simulink model "h16k_ver112c_1500"  (R2012b)
settings: Solver=VariableStepDiscrete  SolverMode=SingleTasking  StartTime=0.0  StopTime=128000  RelTol=1e-3
undefined symbols (not defined in the file or in its folder): sfp
libraries: xbsIndex_r4 x3386, dspsigops x32, casper_library_misc x23, monroe_library x8, simulink x7, xps_library x6
(part 2 of 28)

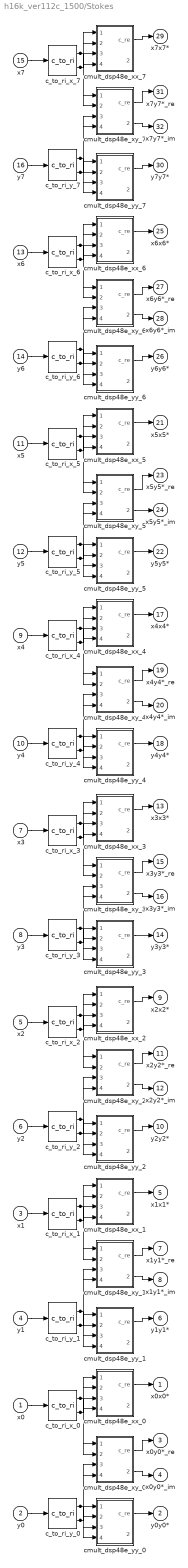
== system h16k_ver112c_1500/Stokes ==
  x0 : Inport
  y0 : Inport  Port=2
  x1 : Inport  Port=3
  y1 : Inport  Port=4
  x2 : Inport  Port=5
  y2 : Inport  Port=6
  x3 : Inport  Port=7
  y3 : Inport  Port=8
  x4 : Inport  Port=9
  y4 : Inport  Port=10
  x5 : Inport  Port=11
  y5 : Inport  Port=12
  x6 : Inport  Port=13
  y6 : Inport  Port=14
  x7 : Inport  Port=15
  y7 : Inport  Port=16
  c_to_ri_x_{0..7} (8 alike) : casper_library_misc/c_to_ri  n_bits=18  bin_pt=0
      settings: AttributesFormatString=18_0 r/i
  c_to_ri_y_{0..7} (8 alike) : casper_library_misc/c_to_ri  n_bits=18  bin_pt=0
      settings: AttributesFormatString=18_0 r/i
  cmult_dsp48e_xx_0 : Subsystem  AncestorBlock=casper_library_multipliers/cmult_dsp48e  mask(cmult_dsp48e){n_bits_a=18, bin_pt_a=0, n_bits_b=18, bin_pt_b=0, conjugated=on, full_precision=on, n_bits_c=37, bin_pt_c=34, quantization=Truncate, overflow=Wrap, cast_latency=0}
      mask prompts: n_bits_a "Bit width 'a'"; bin_pt_a "Binary point 'a'"; n_bits_b "Bit width 'b'"; bin_pt_b "Binary point 'b'"; conjugated "Conjugate"; full_precision "Full precision"; n_bits_c "Bit width out"; bin_pt_c "Binary point out"; cast_latency "Cast Latency"
      mask help:
      | Multiplies two complex numbers using 4 DSP48Es.
      | Conjugation is optional.
      |
      | Re{a} and Im{a} can be up to 25 bits.
      | Re{b} and Im{b} can be up to 18 bits.
      mask init:
      | cmult_dsp48e_init(gcb, ...
      |     'n_bits_a', n_bits_a, ...
      |     'bin_pt_a', bin_pt_a, ...
      |     'n_bits_b', n_bits_b, ...
      |     'bin_pt_b', bin_pt_b, ...
      |     'conjugated', conjugated, ...
      |     'full_precision', full_precision, ...
      |     'n_bits_c', n_bits_c, ...
      |     'bin_pt_c', bin_pt_c, ...
      |     'quantization', quantization, ...
      |     'overflow', overflow, ...
      |     'cast_latency', cast_latency);
      settings: AttributesFormatString=|
      | 18_0 * 18_0 ==> 37_0
      | Latency=4
      mask Callback full_precision:
      | full_precision = get_param(gcb, 'full_precision');
      | 
      | if strcmp(full_precision, 'on'),
      |     not_full_precision = 'off';
      | else
      |     not_full_precision = 'on';
      | end
      | 
      | set_param_state(gcb, 'n_bits_c', not_full_precision);
      | set_param_state(gcb, 'bin_pt_c', not_full_precision);
      | set_param_state(gcb, 'quantization', not_full_precision);
      | set_param_state(gcb, 'overflow', not_full_precision);
      | set_param_state(gcb, 'cast_latency', not_full_precision);
      mask TypeOptions quantization: Truncate | Round  (unbiased: +/- Inf) | Round  (unbiased: Even Values)
      mask TypeOptions overflow: Wrap | Saturate | Flag as error
  cmult_dsp48e_xx_1 : Subsystem  AncestorBlock=casper_library_multipliers/cmult_dsp48e  mask(cmult_dsp48e){n_bits_a=18, bin_pt_a=0, n_bits_b=18, bin_pt_b=0, conjugated=on, full_precision=on, n_bits_c=37, bin_pt_c=34, quantization=Truncate, overflow=Wrap, cast_latency=0}
      mask prompts: n_bits_a "Bit width 'a'"; bin_pt_a "Binary point 'a'"; n_bits_b "Bit width 'b'"; bin_pt_b "Binary point 'b'"; conjugated "Conjugate"; full_precision "Full precision"; n_bits_c "Bit width out"; bin_pt_c "Binary point out"; cast_latency "Cast Latency"
      mask help:
      | Multiplies two complex numbers using 4 DSP48Es.
      | Conjugation is optional.
      |
      | Re{a} and Im{a} can be up to 25 bits.
      | Re{b} and Im{b} can be up to 18 bits.
      mask init: same as h16k_ver112c_1500/Stokes/cmult_dsp48e_xx_0
      settings: AttributesFormatString=|
      | 18_0 * 18_0 ==> 37_0
      | Latency=4
      mask Callback full_precision:
      | full_precision = get_param(gcb, 'full_precision');
      | 
      | if strcmp(full_precision, 'on'),
      |     not_full_precision = 'off';
      | else
      |     not_full_precision = 'on';
      | end
      | 
      | set_param_state(gcb, 'n_bits_c', not_full_precision);
      | set_param_state(gcb, 'bin_pt_c', not_full_precision);
      | set_param_state(gcb, 'quantization', not_full_precision);
      | set_param_state(gcb, 'overflow', not_full_precision);
      | set_param_state(gcb, 'cast_latency', not_full_precision);
      mask TypeOptions quantization: Truncate | Round  (unbiased: +/- Inf) | Round  (unbiased: Even Values)
      mask TypeOptions overflow: Wrap | Saturate | Flag as error
  cmult_dsp48e_xx_2 : Subsystem  AncestorBlock=casper_library_multipliers/cmult_dsp48e  mask(cmult_dsp48e){n_bits_a=18, bin_pt_a=0, n_bits_b=18, bin_pt_b=0, conjugated=on, full_precision=on, n_bits_c=37, bin_pt_c=34, quantization=Truncate, overflow=Wrap, cast_latency=0}
      mask prompts: n_bits_a "Bit width 'a'"; bin_pt_a "Binary point 'a'"; n_bits_b "Bit width 'b'"; bin_pt_b "Binary point 'b'"; conjugated "Conjugate"; full_precision "Full precision"; n_bits_c "Bit width out"; bin_pt_c "Binary point out"; cast_latency "Cast Latency"
      mask help:
      | Multiplies two complex numbers using 4 DSP48Es.
      | Conjugation is optional.
      |
      | Re{a} and Im{a} can be up to 25 bits.
      | Re{b} and Im{b} can be up to 18 bits.
      mask init: same as h16k_ver112c_1500/Stokes/cmult_dsp48e_xx_0
      settings: AttributesFormatString=|
      | 18_0 * 18_0 ==> 37_0
      | Latency=4
      mask Callback full_precision:
      | full_precision = get_param(gcb, 'full_precision');
      | 
      | if strcmp(full_precision, 'on'),
      |     not_full_precision = 'off';
      | else
      |     not_full_precision = 'on';
      | end
      | 
      | set_param_state(gcb, 'n_bits_c', not_full_precision);
      | set_param_state(gcb, 'bin_pt_c', not_full_precision);
      | set_param_state(gcb, 'quantization', not_full_precision);
      | set_param_state(gcb, 'overflow', not_full_precision);
      | set_param_state(gcb, 'cast_latency', not_full_precision);
      mask TypeOptions quantization: Truncate | Round  (unbiased: +/- Inf) | Round  (unbiased: Even Values)
      mask TypeOptions overflow: Wrap | Saturate | Flag as error
  cmult_dsp48e_xx_3 : Subsystem  AncestorBlock=casper_library_multipliers/cmult_dsp48e  mask(cmult_dsp48e){n_bits_a=18, bin_pt_a=0, n_bits_b=18, bin_pt_b=0, conjugated=on, full_precision=on, n_bits_c=37, bin_pt_c=34, quantization=Truncate, overflow=Wrap, cast_latency=0}
      mask prompts: n_bits_a "Bit width 'a'"; bin_pt_a "Binary point 'a'"; n_bits_b "Bit width 'b'"; bin_pt_b "Binary point 'b'"; conjugated "Conjugate"; full_precision "Full precision"; n_bits_c "Bit width out"; bin_pt_c "Binary point out"; cast_latency "Cast Latency"
      mask help:
      | Multiplies two complex numbers using 4 DSP48Es.
      | Conjugation is optional.
      |
      | Re{a} and Im{a} can be up to 25 bits.
      | Re{b} and Im{b} can be up to 18 bits.
      mask init: same as h16k_ver112c_1500/Stokes/cmult_dsp48e_xx_0
      settings: AttributesFormatString=|
      | 18_0 * 18_0 ==> 37_0
      | Latency=4
      mask Callback full_precision:
      | full_precision = get_param(gcb, 'full_precision');
      | 
      | if strcmp(full_precision, 'on'),
      |     not_full_precision = 'off';
      | else
      |     not_full_precision = 'on';
      | end
      | 
      | set_param_state(gcb, 'n_bits_c', not_full_precision);
      | set_param_state(gcb, 'bin_pt_c', not_full_precision);
      | set_param_state(gcb, 'quantization', not_full_precision);
      | set_param_state(gcb, 'overflow', not_full_precision);
      | set_param_state(gcb, 'cast_latency', not_full_precision);
      mask TypeOptions quantization: Truncate | Round  (unbiased: +/- Inf) | Round  (unbiased: Even Values)
      mask TypeOptions overflow: Wrap | Saturate | Flag as error
  cmult_dsp48e_xx_4 : Subsystem  AncestorBlock=casper_library_multipliers/cmult_dsp48e  mask(cmult_dsp48e){n_bits_a=18, bin_pt_a=0, n_bits_b=18, bin_pt_b=0, conjugated=on, full_precision=on, n_bits_c=37, bin_pt_c=34, quantization=Truncate, overflow=Wrap, cast_latency=0}
      mask prompts: n_bits_a "Bit width 'a'"; bin_pt_a "Binary point 'a'"; n_bits_b "Bit width 'b'"; bin_pt_b "Binary point 'b'"; conjugated "Conjugate"; full_precision "Full precision"; n_bits_c "Bit width out"; bin_pt_c "Binary point out"; cast_latency "Cast Latency"
      mask help:
      | Multiplies two complex numbers using 4 DSP48Es.
      | Conjugation is optional.
      |
      | Re{a} and Im{a} can be up to 25 bits.
      | Re{b} and Im{b} can be up to 18 bits.
      mask init: same as h16k_ver112c_1500/Stokes/cmult_dsp48e_xx_0
      settings: AttributesFormatString=|
      | 18_0 * 18_0 ==> 37_0
      | Latency=4
      mask Callback full_precision:
      | full_precision = get_param(gcb, 'full_precision');
      | 
      | if strcmp(full_precision, 'on'),
      |     not_full_precision = 'off';
      | else
      |     not_full_precision = 'on';
      | end
      | 
      | set_param_state(gcb, 'n_bits_c', not_full_precision);
      | set_param_state(gcb, 'bin_pt_c', not_full_precision);
      | set_param_state(gcb, 'quantization', not_full_precision);
      | set_param_state(gcb, 'overflow', not_full_precision);
      | set_param_state(gcb, 'cast_latency', not_full_precision);
      mask TypeOptions quantization: Truncate | Round  (unbiased: +/- Inf) | Round  (unbiased: Even Values)
      mask TypeOptions overflow: Wrap | Saturate | Flag as error
  cmult_dsp48e_xx_5 : Subsystem  AncestorBlock=casper_library_multipliers/cmult_dsp48e  mask(cmult_dsp48e){n_bits_a=18, bin_pt_a=0, n_bits_b=18, bin_pt_b=0, conjugated=on, full_precision=on, n_bits_c=37, bin_pt_c=34, quantization=Truncate, overflow=Wrap, cast_latency=0}
      mask prompts: n_bits_a "Bit width 'a'"; bin_pt_a "Binary point 'a'"; n_bits_b "Bit width 'b'"; bin_pt_b "Binary point 'b'"; conjugated "Conjugate"; full_precision "Full precision"; n_bits_c "Bit width out"; bin_pt_c "Binary point out"; cast_latency "Cast Latency"
      mask help:
      | Multiplies two complex numbers using 4 DSP48Es.
      | Conjugation is optional.
      |
      | Re{a} and Im{a} can be up to 25 bits.
      | Re{b} and Im{b} can be up to 18 bits.
      mask init: same as h16k_ver112c_1500/Stokes/cmult_dsp48e_xx_0
      settings: AttributesFormatString=|
      | 18_0 * 18_0 ==> 37_0
      | Latency=4
      mask Callback full_precision:
      | full_precision = get_param(gcb, 'full_precision');
      | 
      | if strcmp(full_precision, 'on'),
      |     not_full_precision = 'off';
      | else
      |     not_full_precision = 'on';
      | end
      | 
      | set_param_state(gcb, 'n_bits_c', not_full_precision);
      | set_param_state(gcb, 'bin_pt_c', not_full_precision);
      | set_param_state(gcb, 'quantization', not_full_precision);
      | set_param_state(gcb, 'overflow', not_full_precision);
      | set_param_state(gcb, 'cast_latency', not_full_precision);
      mask TypeOptions quantization: Truncate | Round  (unbiased: +/- Inf) | Round  (unbiased: Even Values)
      mask TypeOptions overflow: Wrap | Saturate | Flag as error
  cmult_dsp48e_xx_6 : Subsystem  AncestorBlock=casper_library_multipliers/cmult_dsp48e  mask(cmult_dsp48e){n_bits_a=18, bin_pt_a=0, n_bits_b=18, bin_pt_b=0, conjugated=on, full_precision=on, n_bits_c=37, bin_pt_c=34, quantization=Truncate, overflow=Wrap, cast_latency=0}
      mask prompts: n_bits_a "Bit width 'a'"; bin_pt_a "Binary point 'a'"; n_bits_b "Bit width 'b'"; bin_pt_b "Binary point 'b'"; conjugated "Conjugate"; full_precision "Full precision"; n_bits_c "Bit width out"; bin_pt_c "Binary point out"; cast_latency "Cast Latency"
      mask help:
      | Multiplies two complex numbers using 4 DSP48Es.
      | Conjugation is optional.
      |
      | Re{a} and Im{a} can be up to 25 bits.
      | Re{b} and Im{b} can be up to 18 bits.
      mask init: same as h16k_ver112c_1500/Stokes/cmult_dsp48e_xx_0
      settings: AttributesFormatString=|
      | 18_0 * 18_0 ==> 37_0
      | Latency=4
      mask Callback full_precision:
      | full_precision = get_param(gcb, 'full_precision');
      | 
      | if strcmp(full_precision, 'on'),
      |     not_full_precision = 'off';
      | else
      |     not_full_precision = 'on';
      | end
      | 
      | set_param_state(gcb, 'n_bits_c', not_full_precision);
      | set_param_state(gcb, 'bin_pt_c', not_full_precision);
      | set_param_state(gcb, 'quantization', not_full_precision);
      | set_param_state(gcb, 'overflow', not_full_precision);
      | set_param_state(gcb, 'cast_latency', not_full_precision);
      mask TypeOptions quantization: Truncate | Round  (unbiased: +/- Inf) | Round  (unbiased: Even Values)
      mask TypeOptions overflow: Wrap | Saturate | Flag as error
  cmult_dsp48e_xx_7 : Subsystem  AncestorBlock=casper_library_multipliers/cmult_dsp48e  mask(cmult_dsp48e){n_bits_a=18, bin_pt_a=0, n_bits_b=18, bin_pt_b=0, conjugated=on, full_precision=on, n_bits_c=37, bin_pt_c=34, quantization=Truncate, overflow=Wrap, cast_latency=0}
      mask prompts: n_bits_a "Bit width 'a'"; bin_pt_a "Binary point 'a'"; n_bits_b "Bit width 'b'"; bin_pt_b "Binary point 'b'"; conjugated "Conjugate"; full_precision "Full precision"; n_bits_c "Bit width out"; bin_pt_c "Binary point out"; cast_latency "Cast Latency"
      mask help:
      | Multiplies two complex numbers using 4 DSP48Es.
      | Conjugation is optional.
      |
      | Re{a} and Im{a} can be up to 25 bits.
      | Re{b} and Im{b} can be up to 18 bits.
      mask init: same as h16k_ver112c_1500/Stokes/cmult_dsp48e_xx_0
      settings: AttributesFormatString=|
      | 18_0 * 18_0 ==> 37_0
      | Latency=4
      mask Callback full_precision:
      | full_precision = get_param(gcb, 'full_precision');
      | 
      | if strcmp(full_precision, 'on'),
      |     not_full_precision = 'off';
      | else
      |     not_full_precision = 'on';
      | end
      | 
      | set_param_state(gcb, 'n_bits_c', not_full_precision);
      | set_param_state(gcb, 'bin_pt_c', not_full_precision);
      | set_param_state(gcb, 'quantization', not_full_precision);
      | set_param_state(gcb, 'overflow', not_full_precision);
      | set_param_state(gcb, 'cast_latency', not_full_precision);
      mask TypeOptions quantization: Truncate | Round  (unbiased: +/- Inf) | Round  (unbiased: Even Values)
      mask TypeOptions overflow: Wrap | Saturate | Flag as error
  cmult_dsp48e_xy_0 : Subsystem  AncestorBlock=casper_library_multipliers/cmult_dsp48e  mask(cmult_dsp48e){n_bits_a=18, bin_pt_a=0, n_bits_b=18, bin_pt_b=0, conjugated=on, full_precision=on, n_bits_c=37, bin_pt_c=34, quantization=Truncate, overflow=Wrap, cast_latency=0}
      mask prompts: n_bits_a "Bit width 'a'"; bin_pt_a "Binary point 'a'"; n_bits_b "Bit width 'b'"; bin_pt_b "Binary point 'b'"; conjugated "Conjugate"; full_precision "Full precision"; n_bits_c "Bit width out"; bin_pt_c "Binary point out"; cast_latency "Cast Latency"
      mask help:
      | Multiplies two complex numbers using 4 DSP48Es.
      | Conjugation is optional.
      |
      | Re{a} and Im{a} can be up to 25 bits.
      | Re{b} and Im{b} can be up to 18 bits.
      mask init: same as h16k_ver112c_1500/Stokes/cmult_dsp48e_xx_0
      settings: AttributesFormatString=|
      | 18_0 * 18_0 ==> 37_0
      | Latency=4
      mask Callback full_precision:
      | full_precision = get_param(gcb, 'full_precision');
      | 
      | if strcmp(full_precision, 'on'),
      |     not_full_precision = 'off';
      | else
      |     not_full_precision = 'on';
      | end
      | 
      | set_param_state(gcb, 'n_bits_c', not_full_precision);
      | set_param_state(gcb, 'bin_pt_c', not_full_precision);
      | set_param_state(gcb, 'quantization', not_full_precision);
      | set_param_state(gcb, 'overflow', not_full_precision);
      | set_param_state(gcb, 'cast_latency', not_full_precision);
      mask TypeOptions quantization: Truncate | Round  (unbiased: +/- Inf) | Round  (unbiased: Even Values)
      mask TypeOptions overflow: Wrap | Saturate | Flag as error
  cmult_dsp48e_xy_1 : Subsystem  AncestorBlock=casper_library_multipliers/cmult_dsp48e  mask(cmult_dsp48e){n_bits_a=18, bin_pt_a=0, n_bits_b=18, bin_pt_b=0, conjugated=on, full_precision=on, n_bits_c=37, bin_pt_c=34, quantization=Truncate, overflow=Wrap, cast_latency=0}
      mask prompts: n_bits_a "Bit width 'a'"; bin_pt_a "Binary point 'a'"; n_bits_b "Bit width 'b'"; bin_pt_b "Binary point 'b'"; conjugated "Conjugate"; full_precision "Full precision"; n_bits_c "Bit width out"; bin_pt_c "Binary point out"; cast_latency "Cast Latency"
      mask help:
      | Multiplies two complex numbers using 4 DSP48Es.
      | Conjugation is optional.
      |
      | Re{a} and Im{a} can be up to 25 bits.
      | Re{b} and Im{b} can be up to 18 bits.
      mask init: same as h16k_ver112c_1500/Stokes/cmult_dsp48e_xx_0
      settings: AttributesFormatString=|
      | 18_0 * 18_0 ==> 37_0
      | Latency=4
      mask Callback full_precision:
      | full_precision = get_param(gcb, 'full_precision');
      | 
      | if strcmp(full_precision, 'on'),
      |     not_full_precision = 'off';
      | else
      |     not_full_precision = 'on';
      | end
      | 
      | set_param_state(gcb, 'n_bits_c', not_full_precision);
      | set_param_state(gcb, 'bin_pt_c', not_full_precision);
      | set_param_state(gcb, 'quantization', not_full_precision);
      | set_param_state(gcb, 'overflow', not_full_precision);
      | set_param_state(gcb, 'cast_latency', not_full_precision);
      mask TypeOptions quantization: Truncate | Round  (unbiased: +/- Inf) | Round  (unbiased: Even Values)
      mask TypeOptions overflow: Wrap | Saturate | Flag as error
  cmult_dsp48e_xy_2 : Subsystem  AncestorBlock=casper_library_multipliers/cmult_dsp48e  mask(cmult_dsp48e){n_bits_a=18, bin_pt_a=0, n_bits_b=18, bin_pt_b=0, conjugated=on, full_precision=on, n_bits_c=37, bin_pt_c=34, quantization=Truncate, overflow=Wrap, cast_latency=0}
      mask prompts: n_bits_a "Bit width 'a'"; bin_pt_a "Binary point 'a'"; n_bits_b "Bit width 'b'"; bin_pt_b "Binary point 'b'"; conjugated "Conjugate"; full_precision "Full precision"; n_bits_c "Bit width out"; bin_pt_c "Binary point out"; cast_latency "Cast Latency"
      mask help:
      | Multiplies two complex numbers using 4 DSP48Es.
      | Conjugation is optional.
      |
      | Re{a} and Im{a} can be up to 25 bits.
      | Re{b} and Im{b} can be up to 18 bits.
      mask init: same as h16k_ver112c_1500/Stokes/cmult_dsp48e_xx_0
      settings: AttributesFormatString=|
      | 18_0 * 18_0 ==> 37_0
      | Latency=4
      mask Callback full_precision:
      | full_precision = get_param(gcb, 'full_precision');
      | 
      | if strcmp(full_precision, 'on'),
      |     not_full_precision = 'off';
      | else
      |     not_full_precision = 'on';
      | end
      | 
      | set_param_state(gcb, 'n_bits_c', not_full_precision);
      | set_param_state(gcb, 'bin_pt_c', not_full_precision);
      | set_param_state(gcb, 'quantization', not_full_precision);
      | set_param_state(gcb, 'overflow', not_full_precision);
      | set_param_state(gcb, 'cast_latency', not_full_precision);
      mask TypeOptions quantization: Truncate | Round  (unbiased: +/- Inf) | Round  (unbiased: Even Values)
      mask TypeOptions overflow: Wrap | Saturate | Flag as error
  cmult_dsp48e_xy_3 : Subsystem  AncestorBlock=casper_library_multipliers/cmult_dsp48e  mask(cmult_dsp48e){n_bits_a=18, bin_pt_a=0, n_bits_b=18, bin_pt_b=0, conjugated=on, full_precision=on, n_bits_c=37, bin_pt_c=34, quantization=Truncate, overflow=Wrap, cast_latency=0}
      mask prompts: n_bits_a "Bit width 'a'"; bin_pt_a "Binary point 'a'"; n_bits_b "Bit width 'b'"; bin_pt_b "Binary point 'b'"; conjugated "Conjugate"; full_precision "Full precision"; n_bits_c "Bit width out"; bin_pt_c "Binary point out"; cast_latency "Cast Latency"
      mask help:
      | Multiplies two complex numbers using 4 DSP48Es.
      | Conjugation is optional.
      |
      | Re{a} and Im{a} can be up to 25 bits.
      | Re{b} and Im{b} can be up to 18 bits.
      mask init: same as h16k_ver112c_1500/Stokes/cmult_dsp48e_xx_0
      settings: AttributesFormatString=|
      | 18_0 * 18_0 ==> 37_0
      | Latency=4
      mask Callback full_precision:
      | full_precision = get_param(gcb, 'full_precision');
      | 
      | if strcmp(full_precision, 'on'),
      |     not_full_precision = 'off';
      | else
      |     not_full_precision = 'on';
      | end
      | 
      | set_param_state(gcb, 'n_bits_c', not_full_precision);
      | set_param_state(gcb, 'bin_pt_c', not_full_precision);
      | set_param_state(gcb, 'quantization', not_full_precision);
      | set_param_state(gcb, 'overflow', not_full_precision);
      | set_param_state(gcb, 'cast_latency', not_full_precision);
      mask TypeOptions quantization: Truncate | Round  (unbiased: +/- Inf) | Round  (unbiased: Even Values)
      mask TypeOptions overflow: Wrap | Saturate | Flag as error
  cmult_dsp48e_xy_4 : Subsystem  AncestorBlock=casper_library_multipliers/cmult_dsp48e  mask(cmult_dsp48e){n_bits_a=18, bin_pt_a=0, n_bits_b=18, bin_pt_b=0, conjugated=on, full_precision=on, n_bits_c=37, bin_pt_c=34, quantization=Truncate, overflow=Wrap, cast_latency=0}
      mask prompts: n_bits_a "Bit width 'a'"; bin_pt_a "Binary point 'a'"; n_bits_b "Bit width 'b'"; bin_pt_b "Binary point 'b'"; conjugated "Conjugate"; full_precision "Full precision"; n_bits_c "Bit width out"; bin_pt_c "Binary point out"; cast_latency "Cast Latency"
      mask help:
      | Multiplies two complex numbers using 4 DSP48Es.
      | Conjugation is optional.
      |
      | Re{a} and Im{a} can be up to 25 bits.
      | Re{b} and Im{b} can be up to 18 bits.
      mask init: same as h16k_ver112c_1500/Stokes/cmult_dsp48e_xx_0
      settings: AttributesFormatString=|
      | 18_0 * 18_0 ==> 37_0
      | Latency=4
      mask Callback full_precision:
      | full_precision = get_param(gcb, 'full_precision');
      | 
      | if strcmp(full_precision, 'on'),
      |     not_full_precision = 'off';
      | else
      |     not_full_precision = 'on';
      | end
      | 
      | set_param_state(gcb, 'n_bits_c', not_full_precision);
      | set_param_state(gcb, 'bin_pt_c', not_full_precision);
      | set_param_state(gcb, 'quantization', not_full_precision);
      | set_param_state(gcb, 'overflow', not_full_precision);
      | set_param_state(gcb, 'cast_latency', not_full_precision);
      mask TypeOptions quantization: Truncate | Round  (unbiased: +/- Inf) | Round  (unbiased: Even Values)
      mask TypeOptions overflow: Wrap | Saturate | Flag as error
  cmult_dsp48e_xy_5 : Subsystem  AncestorBlock=casper_library_multipliers/cmult_dsp48e  mask(cmult_dsp48e){n_bits_a=18, bin_pt_a=0, n_bits_b=18, bin_pt_b=0, conjugated=on, full_precision=on, n_bits_c=37, bin_pt_c=34, quantization=Truncate, overflow=Wrap, cast_latency=0}
      mask prompts: n_bits_a "Bit width 'a'"; bin_pt_a "Binary point 'a'"; n_bits_b "Bit width 'b'"; bin_pt_b "Binary point 'b'"; conjugated "Conjugate"; full_precision "Full precision"; n_bits_c "Bit width out"; bin_pt_c "Binary point out"; cast_latency "Cast Latency"
      mask help:
      | Multiplies two complex numbers using 4 DSP48Es.
      | Conjugation is optional.
      |
      | Re{a} and Im{a} can be up to 25 bits.
      | Re{b} and Im{b} can be up to 18 bits.
      mask init: same as h16k_ver112c_1500/Stokes/cmult_dsp48e_xx_0
      settings: AttributesFormatString=|
      | 18_0 * 18_0 ==> 37_0
      | Latency=4
      mask Callback full_precision:
      | full_precision = get_param(gcb, 'full_precision');
      | 
      | if strcmp(full_precision, 'on'),
      |     not_full_precision = 'off';
      | else
      |     not_full_precision = 'on';
      | end
      | 
      | set_param_state(gcb, 'n_bits_c', not_full_precision);
      | set_param_state(gcb, 'bin_pt_c', not_full_precision);
      | set_param_state(gcb, 'quantization', not_full_precision);
      | set_param_state(gcb, 'overflow', not_full_precision);
      | set_param_state(gcb, 'cast_latency', not_full_precision);
      mask TypeOptions quantization: Truncate | Round  (unbiased: +/- Inf) | Round  (unbiased: Even Values)
      mask TypeOptions overflow: Wrap | Saturate | Flag as error
  cmult_dsp48e_xy_6 : Subsystem  AncestorBlock=casper_library_multipliers/cmult_dsp48e  mask(cmult_dsp48e){n_bits_a=18, bin_pt_a=0, n_bits_b=18, bin_pt_b=0, conjugated=on, full_precision=on, n_bits_c=37, bin_pt_c=34, quantization=Truncate, overflow=Wrap, cast_latency=0}
      mask prompts: n_bits_a "Bit width 'a'"; bin_pt_a "Binary point 'a'"; n_bits_b "Bit width 'b'"; bin_pt_b "Binary point 'b'"; conjugated "Conjugate"; full_precision "Full precision"; n_bits_c "Bit width out"; bin_pt_c "Binary point out"; cast_latency "Cast Latency"
      mask help:
      | Multiplies two complex numbers using 4 DSP48Es.
      | Conjugation is optional.
      |
      | Re{a} and Im{a} can be up to 25 bits.
      | Re{b} and Im{b} can be up to 18 bits.
      mask init: same as h16k_ver112c_1500/Stokes/cmult_dsp48e_xx_0
      settings: AttributesFormatString=|
      | 18_0 * 18_0 ==> 37_0
      | Latency=4
      mask Callback full_precision:
      | full_precision = get_param(gcb, 'full_precision');
      | 
      | if strcmp(full_precision, 'on'),
      |     not_full_precision = 'off';
      | else
      |     not_full_precision = 'on';
      | end
      | 
      | set_param_state(gcb, 'n_bits_c', not_full_precision);
      | set_param_state(gcb, 'bin_pt_c', not_full_precision);
      | set_param_state(gcb, 'quantization', not_full_precision);
      | set_param_state(gcb, 'overflow', not_full_precision);
      | set_param_state(gcb, 'cast_latency', not_full_precision);
      mask TypeOptions quantization: Truncate | Round  (unbiased: +/- Inf) | Round  (unbiased: Even Values)
      mask TypeOptions overflow: Wrap | Saturate | Flag as error
  cmult_dsp48e_xy_7 : Subsystem  AncestorBlock=casper_library_multipliers/cmult_dsp48e  mask(cmult_dsp48e){n_bits_a=18, bin_pt_a=0, n_bits_b=18, bin_pt_b=0, conjugated=on, full_precision=on, n_bits_c=37, bin_pt_c=34, quantization=Truncate, overflow=Wrap, cast_latency=0}
      mask prompts: n_bits_a "Bit width 'a'"; bin_pt_a "Binary point 'a'"; n_bits_b "Bit width 'b'"; bin_pt_b "Binary point 'b'"; conjugated "Conjugate"; full_precision "Full precision"; n_bits_c "Bit width out"; bin_pt_c "Binary point out"; cast_latency "Cast Latency"
      mask help:
      | Multiplies two complex numbers using 4 DSP48Es.
      | Conjugation is optional.
      |
      | Re{a} and Im{a} can be up to 25 bits.
      | Re{b} and Im{b} can be up to 18 bits.
      mask init: same as h16k_ver112c_1500/Stokes/cmult_dsp48e_xx_0
      settings: AttributesFormatString=|
      | 18_0 * 18_0 ==> 37_0
      | Latency=4
      mask Callback full_precision:
      | full_precision = get_param(gcb, 'full_precision');
      | 
      | if strcmp(full_precision, 'on'),
      |     not_full_precision = 'off';
      | else
      |     not_full_precision = 'on';
      | end
      | 
      | set_param_state(gcb, 'n_bits_c', not_full_precision);
      | set_param_state(gcb, 'bin_pt_c', not_full_precision);
      | set_param_state(gcb, 'quantization', not_full_precision);
      | set_param_state(gcb, 'overflow', not_full_precision);
      | set_param_state(gcb, 'cast_latency', not_full_precision);
      mask TypeOptions quantization: Truncate | Round  (unbiased: +/- Inf) | Round  (unbiased: Even Values)
      mask TypeOptions overflow: Wrap | Saturate | Flag as error
  cmult_dsp48e_yy_0 : Subsystem  AncestorBlock=casper_library_multipliers/cmult_dsp48e  mask(cmult_dsp48e){n_bits_a=18, bin_pt_a=0, n_bits_b=18, bin_pt_b=0, conjugated=on, full_precision=on, n_bits_c=37, bin_pt_c=34, quantization=Truncate, overflow=Wrap, cast_latency=0}
      mask prompts: n_bits_a "Bit width 'a'"; bin_pt_a "Binary point 'a'"; n_bits_b "Bit width 'b'"; bin_pt_b "Binary point 'b'"; conjugated "Conjugate"; full_precision "Full precision"; n_bits_c "Bit width out"; bin_pt_c "Binary point out"; cast_latency "Cast Latency"
      mask help:
      | Multiplies two complex numbers using 4 DSP48Es.
      | Conjugation is optional.
      |
      | Re{a} and Im{a} can be up to 25 bits.
      | Re{b} and Im{b} can be up to 18 bits.
      mask init: same as h16k_ver112c_1500/Stokes/cmult_dsp48e_xx_0
      settings: AttributesFormatString=|
      | 18_0 * 18_0 ==> 37_0
      | Latency=4
      mask Callback full_precision:
      | full_precision = get_param(gcb, 'full_precision');
      | 
      | if strcmp(full_precision, 'on'),
      |     not_full_precision = 'off';
      | else
      |     not_full_precision = 'on';
      | end
      | 
      | set_param_state(gcb, 'n_bits_c', not_full_precision);
      | set_param_state(gcb, 'bin_pt_c', not_full_precision);
      | set_param_state(gcb, 'quantization', not_full_precision);
      | set_param_state(gcb, 'overflow', not_full_precision);
      | set_param_state(gcb, 'cast_latency', not_full_precision);
      mask TypeOptions quantization: Truncate | Round  (unbiased: +/- Inf) | Round  (unbiased: Even Values)
      mask TypeOptions overflow: Wrap | Saturate | Flag as error
  cmult_dsp48e_yy_1 : Subsystem  AncestorBlock=casper_library_multipliers/cmult_dsp48e  mask(cmult_dsp48e){n_bits_a=18, bin_pt_a=0, n_bits_b=18, bin_pt_b=0, conjugated=on, full_precision=on, n_bits_c=37, bin_pt_c=34, quantization=Truncate, overflow=Wrap, cast_latency=0}
      mask prompts: n_bits_a "Bit width 'a'"; bin_pt_a "Binary point 'a'"; n_bits_b "Bit width 'b'"; bin_pt_b "Binary point 'b'"; conjugated "Conjugate"; full_precision "Full precision"; n_bits_c "Bit width out"; bin_pt_c "Binary point out"; cast_latency "Cast Latency"
      mask help:
      | Multiplies two complex numbers using 4 DSP48Es.
      | Conjugation is optional.
      |
      | Re{a} and Im{a} can be up to 25 bits.
      | Re{b} and Im{b} can be up to 18 bits.
      mask init: same as h16k_ver112c_1500/Stokes/cmult_dsp48e_xx_0
      settings: AttributesFormatString=|
      | 18_0 * 18_0 ==> 37_0
      | Latency=4
      mask Callback full_precision:
      | full_precision = get_param(gcb, 'full_precision');
      | 
      | if strcmp(full_precision, 'on'),
      |     not_full_precision = 'off';
      | else
      |     not_full_precision = 'on';
      | end
      | 
      | set_param_state(gcb, 'n_bits_c', not_full_precision);
      | set_param_state(gcb, 'bin_pt_c', not_full_precision);
      | set_param_state(gcb, 'quantization', not_full_precision);
      | set_param_state(gcb, 'overflow', not_full_precision);
      | set_param_state(gcb, 'cast_latency', not_full_precision);
      mask TypeOptions quantization: Truncate | Round  (unbiased: +/- Inf) | Round  (unbiased: Even Values)
      mask TypeOptions overflow: Wrap | Saturate | Flag as error
  cmult_dsp48e_yy_2 : Subsystem  AncestorBlock=casper_library_multipliers/cmult_dsp48e  mask(cmult_dsp48e){n_bits_a=18, bin_pt_a=0, n_bits_b=18, bin_pt_b=0, conjugated=on, full_precision=on, n_bits_c=37, bin_pt_c=34, quantization=Truncate, overflow=Wrap, cast_latency=0}
      mask prompts: n_bits_a "Bit width 'a'"; bin_pt_a "Binary point 'a'"; n_bits_b "Bit width 'b'"; bin_pt_b "Binary point 'b'"; conjugated "Conjugate"; full_precision "Full precision"; n_bits_c "Bit width out"; bin_pt_c "Binary point out"; cast_latency "Cast Latency"
      mask help:
      | Multiplies two complex numbers using 4 DSP48Es.
      | Conjugation is optional.
      |
      | Re{a} and Im{a} can be up to 25 bits.
      | Re{b} and Im{b} can be up to 18 bits.
      mask init: same as h16k_ver112c_1500/Stokes/cmult_dsp48e_xx_0
      settings: AttributesFormatString=|
      | 18_0 * 18_0 ==> 37_0
      | Latency=4
      mask Callback full_precision:
      | full_precision = get_param(gcb, 'full_precision');
      | 
      | if strcmp(full_precision, 'on'),
      |     not_full_precision = 'off';
      | else
      |     not_full_precision = 'on';
      | end
      | 
      | set_param_state(gcb, 'n_bits_c', not_full_precision);
      | set_param_state(gcb, 'bin_pt_c', not_full_precision);
      | set_param_state(gcb, 'quantization', not_full_precision);
      | set_param_state(gcb, 'overflow', not_full_precision);
      | set_param_state(gcb, 'cast_latency', not_full_precision);
      mask TypeOptions quantization: Truncate | Round  (unbiased: +/- Inf) | Round  (unbiased: Even Values)
      mask TypeOptions overflow: Wrap | Saturate | Flag as error
  cmult_dsp48e_yy_3 : Subsystem  AncestorBlock=casper_library_multipliers/cmult_dsp48e  mask(cmult_dsp48e){n_bits_a=18, bin_pt_a=0, n_bits_b=18, bin_pt_b=0, conjugated=on, full_precision=on, n_bits_c=37, bin_pt_c=34, quantization=Truncate, overflow=Wrap, cast_latency=0}
      mask prompts: n_bits_a "Bit width 'a'"; bin_pt_a "Binary point 'a'"; n_bits_b "Bit width 'b'"; bin_pt_b "Binary point 'b'"; conjugated "Conjugate"; full_precision "Full precision"; n_bits_c "Bit width out"; bin_pt_c "Binary point out"; cast_latency "Cast Latency"
      mask help:
      | Multiplies two complex numbers using 4 DSP48Es.
      | Conjugation is optional.
      |
      | Re{a} and Im{a} can be up to 25 bits.
      | Re{b} and Im{b} can be up to 18 bits.
      mask init: same as h16k_ver112c_1500/Stokes/cmult_dsp48e_xx_0
      settings: AttributesFormatString=|
      | 18_0 * 18_0 ==> 37_0
      | Latency=4
      mask Callback full_precision:
      | full_precision = get_param(gcb, 'full_precision');
      | 
      | if strcmp(full_precision, 'on'),
      |     not_full_precision = 'off';
      | else
      |     not_full_precision = 'on';
      | end
      | 
      | set_param_state(gcb, 'n_bits_c', not_full_precision);
      | set_param_state(gcb, 'bin_pt_c', not_full_precision);
      | set_param_state(gcb, 'quantization', not_full_precision);
      | set_param_state(gcb, 'overflow', not_full_precision);
      | set_param_state(gcb, 'cast_latency', not_full_precision);
      mask TypeOptions quantization: Truncate | Round  (unbiased: +/- Inf) | Round  (unbiased: Even Values)
      mask TypeOptions overflow: Wrap | Saturate | Flag as error
  cmult_dsp48e_yy_4 : Subsystem  AncestorBlock=casper_library_multipliers/cmult_dsp48e  mask(cmult_dsp48e){n_bits_a=18, bin_pt_a=0, n_bits_b=18, bin_pt_b=0, conjugated=on, full_precision=on, n_bits_c=37, bin_pt_c=34, quantization=Truncate, overflow=Wrap, cast_latency=0}
      mask prompts: n_bits_a "Bit width 'a'"; bin_pt_a "Binary point 'a'"; n_bits_b "Bit width 'b'"; bin_pt_b "Binary point 'b'"; conjugated "Conjugate"; full_precision "Full precision"; n_bits_c "Bit width out"; bin_pt_c "Binary point out"; cast_latency "Cast Latency"
      mask help:
      | Multiplies two complex numbers using 4 DSP48Es.
      | Conjugation is optional.
      |
      | Re{a} and Im{a} can be up to 25 bits.
      | Re{b} and Im{b} can be up to 18 bits.
      mask init: same as h16k_ver112c_1500/Stokes/cmult_dsp48e_xx_0
      settings: AttributesFormatString=|
      | 18_0 * 18_0 ==> 37_0
      | Latency=4
      mask Callback full_precision:
      | full_precision = get_param(gcb, 'full_precision');
      | 
      | if strcmp(full_precision, 'on'),
      |     not_full_precision = 'off';
      | else
      |     not_full_precision = 'on';
      | end
      | 
      | set_param_state(gcb, 'n_bits_c', not_full_precision);
      | set_param_state(gcb, 'bin_pt_c', not_full_precision);
      | set_param_state(gcb, 'quantization', not_full_precision);
      | set_param_state(gcb, 'overflow', not_full_precision);
      | set_param_state(gcb, 'cast_latency', not_full_precision);
      mask TypeOptions quantization: Truncate | Round  (unbiased: +/- Inf) | Round  (unbiased: Even Values)
      mask TypeOptions overflow: Wrap | Saturate | Flag as error
  cmult_dsp48e_yy_5 : Subsystem  AncestorBlock=casper_library_multipliers/cmult_dsp48e  mask(cmult_dsp48e){n_bits_a=18, bin_pt_a=0, n_bits_b=18, bin_pt_b=0, conjugated=on, full_precision=on, n_bits_c=37, bin_pt_c=34, quantization=Truncate, overflow=Wrap, cast_latency=0}
      mask prompts: n_bits_a "Bit width 'a'"; bin_pt_a "Binary point 'a'"; n_bits_b "Bit width 'b'"; bin_pt_b "Binary point 'b'"; conjugated "Conjugate"; full_precision "Full precision"; n_bits_c "Bit width out"; bin_pt_c "Binary point out"; cast_latency "Cast Latency"
      mask help:
      | Multiplies two complex numbers using 4 DSP48Es.
      | Conjugation is optional.
      |
      | Re{a} and Im{a} can be up to 25 bits.
      | Re{b} and Im{b} can be up to 18 bits.
      mask init: same as h16k_ver112c_1500/Stokes/cmult_dsp48e_xx_0
      settings: AttributesFormatString=|
      | 18_0 * 18_0 ==> 37_0
      | Latency=4
      mask Callback full_precision:
      | full_precision = get_param(gcb, 'full_precision');
      | 
      | if strcmp(full_precision, 'on'),
      |     not_full_precision = 'off';
      | else
      |     not_full_precision = 'on';
      | end
      | 
      | set_param_state(gcb, 'n_bits_c', not_full_precision);
      | set_param_state(gcb, 'bin_pt_c', not_full_precision);
      | set_param_state(gcb, 'quantization', not_full_precision);
      | set_param_state(gcb, 'overflow', not_full_precision);
      | set_param_state(gcb, 'cast_latency', not_full_precision);
      mask TypeOptions quantization: Truncate | Round  (unbiased: +/- Inf) | Round  (unbiased: Even Values)
      mask TypeOptions overflow: Wrap | Saturate | Flag as error
  cmult_dsp48e_yy_6 : Subsystem  AncestorBlock=casper_library_multipliers/cmult_dsp48e  mask(cmult_dsp48e){n_bits_a=18, bin_pt_a=0, n_bits_b=18, bin_pt_b=0, conjugated=on, full_precision=on, n_bits_c=37, bin_pt_c=34, quantization=Truncate, overflow=Wrap, cast_latency=0}
      mask prompts: n_bits_a "Bit width 'a'"; bin_pt_a "Binary point 'a'"; n_bits_b "Bit width 'b'"; bin_pt_b "Binary point 'b'"; conjugated "Conjugate"; full_precision "Full precision"; n_bits_c "Bit width out"; bin_pt_c "Binary point out"; cast_latency "Cast Latency"
      mask help:
      | Multiplies two complex numbers using 4 DSP48Es.
      | Conjugation is optional.
      |
      | Re{a} and Im{a} can be up to 25 bits.
      | Re{b} and Im{b} can be up to 18 bits.
      mask init: same as h16k_ver112c_1500/Stokes/cmult_dsp48e_xx_0
      settings: AttributesFormatString=|
      | 18_0 * 18_0 ==> 37_0
      | Latency=4
      mask Callback full_precision:
      | full_precision = get_param(gcb, 'full_precision');
      | 
      | if strcmp(full_precision, 'on'),
      |     not_full_precision = 'off';
      | else
      |     not_full_precision = 'on';
      | end
      | 
      | set_param_state(gcb, 'n_bits_c', not_full_precision);
      | set_param_state(gcb, 'bin_pt_c', not_full_precision);
      | set_param_state(gcb, 'quantization', not_full_precision);
      | set_param_state(gcb, 'overflow', not_full_precision);
      | set_param_state(gcb, 'cast_latency', not_full_precision);
      mask TypeOptions quantization: Truncate | Round  (unbiased: +/- Inf) | Round  (unbiased: Even Values)
      mask TypeOptions overflow: Wrap | Saturate | Flag as error
  cmult_dsp48e_yy_7 : Subsystem  AncestorBlock=casper_library_multipliers/cmult_dsp48e  mask(cmult_dsp48e){n_bits_a=18, bin_pt_a=0, n_bits_b=18, bin_pt_b=0, conjugated=on, full_precision=on, n_bits_c=37, bin_pt_c=34, quantization=Truncate, overflow=Wrap, cast_latency=0}
      mask prompts: n_bits_a "Bit width 'a'"; bin_pt_a "Binary point 'a'"; n_bits_b "Bit width 'b'"; bin_pt_b "Binary point 'b'"; conjugated "Conjugate"; full_precision "Full precision"; n_bits_c "Bit width out"; bin_pt_c "Binary point out"; cast_latency "Cast Latency"
      mask help:
      | Multiplies two complex numbers using 4 DSP48Es.
      | Conjugation is optional.
      |
      | Re{a} and Im{a} can be up to 25 bits.
      | Re{b} and Im{b} can be up to 18 bits.
      mask init: same as h16k_ver112c_1500/Stokes/cmult_dsp48e_xx_0
      settings: AttributesFormatString=|
      | 18_0 * 18_0 ==> 37_0
      | Latency=4
      mask Callback full_precision:
      | full_precision = get_param(gcb, 'full_precision');
      | 
      | if strcmp(full_precision, 'on'),
      |     not_full_precision = 'off';
      | else
      |     not_full_precision = 'on';
      | end
      | 
      | set_param_state(gcb, 'n_bits_c', not_full_precision);
      | set_param_state(gcb, 'bin_pt_c', not_full_precision);
      | set_param_state(gcb, 'quantization', not_full_precision);
      | set_param_state(gcb, 'overflow', not_full_precision);
      | set_param_state(gcb, 'cast_latency', not_full_precision);
      mask TypeOptions quantization: Truncate | Round  (unbiased: +/- Inf) | Round  (unbiased: Even Values)
      mask TypeOptions overflow: Wrap | Saturate | Flag as error
  x0x0* : Outport
  y0y0* : Outport  Port=2
  x0y0*_re : Outport  Port=3
  x0y0*_im : Outport  Port=4
  x1x1* : Outport  Port=5
  y1y1* : Outport  Port=6
  x1y1*_re : Outport  Port=7
  x1y1*_im : Outport  Port=8
  x2x2* : Outport  Port=9
  y2y2* : Outport  Port=10
  x2y2*_re : Outport  Port=11
  x2y2*_im : Outport  Port=12
  x3x3* : Outport  Port=13
  y3y3* : Outport  Port=14
  x3y3*_re : Outport  Port=15
  x3y3*_im : Outport  Port=16
  x4x4* : Outport  Port=17
  y4y4* : Outport  Port=18
  x4y4*_re : Outport  Port=19
  x4y4*_im : Outport  Port=20
  x5x5* : Outport  Port=21
  y5y5* : Outport  Port=22
  x5y5*_re : Outport  Port=23
  x5y5*_im : Outport  Port=24
  x6x6* : Outport  Port=25
  y6y6* : Outport  Port=26
  x6y6*_re : Outport  Port=27
  x6y6*_im : Outport  Port=28
  x7x7* : Outport  Port=29
  y7y7* : Outport  Port=30
  x7y7*_re : Outport  Port=31
  x7y7*_im : Outport  Port=32
  wires:
  c_to_ri_x_0/1 -> cmult_dsp48e_xy_0/1(a_re), cmult_dsp48e_xx_0/3(b_re), cmult_dsp48e_xx_0/1(a_re)
  c_to_ri_x_0/2 -> cmult_dsp48e_xy_0/2(a_im), cmult_dsp48e_xx_0/4(b_im), cmult_dsp48e_xx_0/2(a_im)
  c_to_ri_y_0/1 -> cmult_dsp48e_xy_0/3(b_re), cmult_dsp48e_yy_0/3(b_re), cmult_dsp48e_yy_0/1(a_re)
  c_to_ri_y_0/2 -> cmult_dsp48e_xy_0/4(b_im), cmult_dsp48e_yy_0/4(b_im), cmult_dsp48e_yy_0/2(a_im)
  c_to_ri_x_1/1 -> cmult_dsp48e_xy_1/1(a_re), cmult_dsp48e_xx_1/3(b_re), cmult_dsp48e_xx_1/1(a_re)
  c_to_ri_x_1/2 -> cmult_dsp48e_xy_1/2(a_im), cmult_dsp48e_xx_1/4(b_im), cmult_dsp48e_xx_1/2(a_im)
  c_to_ri_y_1/1 -> cmult_dsp48e_xy_1/3(b_re), cmult_dsp48e_yy_1/3(b_re), cmult_dsp48e_yy_1/1(a_re)
  c_to_ri_y_1/2 -> cmult_dsp48e_xy_1/4(b_im), cmult_dsp48e_yy_1/4(b_im), cmult_dsp48e_yy_1/2(a_im)
  c_to_ri_x_2/1 -> cmult_dsp48e_xy_2/1(a_re), cmult_dsp48e_xx_2/3(b_re), cmult_dsp48e_xx_2/1(a_re)
  c_to_ri_x_2/2 -> cmult_dsp48e_xy_2/2(a_im), cmult_dsp48e_xx_2/4(b_im), cmult_dsp48e_xx_2/2(a_im)
  c_to_ri_y_2/1 -> cmult_dsp48e_xy_2/3(b_re), cmult_dsp48e_yy_2/3(b_re), cmult_dsp48e_yy_2/1(a_re)
  c_to_ri_y_2/2 -> cmult_dsp48e_xy_2/4(b_im), cmult_dsp48e_yy_2/4(b_im), cmult_dsp48e_yy_2/2(a_im)
  c_to_ri_x_3/1 -> cmult_dsp48e_xy_3/1(a_re), cmult_dsp48e_xx_3/3(b_re), cmult_dsp48e_xx_3/1(a_re)
  c_to_ri_x_3/2 -> cmult_dsp48e_xy_3/2(a_im), cmult_dsp48e_xx_3/4(b_im), cmult_dsp48e_xx_3/2(a_im)
  c_to_ri_y_3/1 -> cmult_dsp48e_xy_3/3(b_re), cmult_dsp48e_yy_3/3(b_re), cmult_dsp48e_yy_3/1(a_re)
  c_to_ri_y_3/2 -> cmult_dsp48e_xy_3/4(b_im), cmult_dsp48e_yy_3/4(b_im), cmult_dsp48e_yy_3/2(a_im)
  c_to_ri_x_4/1 -> cmult_dsp48e_xy_4/1(a_re), cmult_dsp48e_xx_4/3(b_re), cmult_dsp48e_xx_4/1(a_re)
  c_to_ri_x_4/2 -> cmult_dsp48e_xy_4/2(a_im), cmult_dsp48e_xx_4/4(b_im), cmult_dsp48e_xx_4/2(a_im)
  c_to_ri_y_4/1 -> cmult_dsp48e_xy_4/3(b_re), cmult_dsp48e_yy_4/3(b_re), cmult_dsp48e_yy_4/1(a_re)
  c_to_ri_y_4/2 -> cmult_dsp48e_xy_4/4(b_im), cmult_dsp48e_yy_4/4(b_im), cmult_dsp48e_yy_4/2(a_im)
  c_to_ri_x_5/1 -> cmult_dsp48e_xy_5/1(a_re), cmult_dsp48e_xx_5/3(b_re), cmult_dsp48e_xx_5/1(a_re)
  c_to_ri_x_5/2 -> cmult_dsp48e_xy_5/2(a_im), cmult_dsp48e_xx_5/4(b_im), cmult_dsp48e_xx_5/2(a_im)
  c_to_ri_y_5/1 -> cmult_dsp48e_xy_5/3(b_re), cmult_dsp48e_yy_5/3(b_re), cmult_dsp48e_yy_5/1(a_re)
  c_to_ri_y_5/2 -> cmult_dsp48e_xy_5/4(b_im), cmult_dsp48e_yy_5/4(b_im), cmult_dsp48e_yy_5/2(a_im)
  c_to_ri_x_6/1 -> cmult_dsp48e_xy_6/1(a_re), cmult_dsp48e_xx_6/3(b_re), cmult_dsp48e_xx_6/1(a_re)
  c_to_ri_x_6/2 -> cmult_dsp48e_xy_6/2(a_im), cmult_dsp48e_xx_6/4(b_im), cmult_dsp48e_xx_6/2(a_im)
  c_to_ri_y_6/1 -> cmult_dsp48e_xy_6/3(b_re), cmult_dsp48e_yy_6/3(b_re), cmult_dsp48e_yy_6/1(a_re)
  c_to_ri_y_6/2 -> cmult_dsp48e_xy_6/4(b_im), cmult_dsp48e_yy_6/4(b_im), cmult_dsp48e_yy_6/2(a_im)
  c_to_ri_x_7/1 -> cmult_dsp48e_xy_7/1(a_re), cmult_dsp48e_xx_7/3(b_re), cmult_dsp48e_xx_7/1(a_re)
  c_to_ri_x_7/2 -> cmult_dsp48e_xy_7/2(a_im), cmult_dsp48e_xx_7/4(b_im), cmult_dsp48e_xx_7/2(a_im)
  c_to_ri_y_7/1 -> cmult_dsp48e_xy_7/3(b_re), cmult_dsp48e_yy_7/3(b_re), cmult_dsp48e_yy_7/1(a_re)
  c_to_ri_y_7/2 -> cmult_dsp48e_xy_7/4(b_im), cmult_dsp48e_yy_7/4(b_im), cmult_dsp48e_yy_7/2(a_im)
  cmult_dsp48e_xy_7/2(c_im) -> x7y7*_im/1
  cmult_dsp48e_xy_7/1(c_re) -> x7y7*_re/1
  cmult_dsp48e_yy_7/1(c_re) -> y7y7*/1
  cmult_dsp48e_xx_7/1(c_re) -> x7x7*/1
  y7/1 -> c_to_ri_y_7/1
  x7/1 -> c_to_ri_x_7/1
  cmult_dsp48e_xy_6/2(c_im) -> x6y6*_im/1
  cmult_dsp48e_xy_6/1(c_re) -> x6y6*_re/1
  cmult_dsp48e_yy_6/1(c_re) -> y6y6*/1
  cmult_dsp48e_xx_6/1(c_re) -> x6x6*/1
  y6/1 -> c_to_ri_y_6/1
  x6/1 -> c_to_ri_x_6/1
  cmult_dsp48e_xy_5/2(c_im) -> x5y5*_im/1
  cmult_dsp48e_xy_5/1(c_re) -> x5y5*_re/1
  cmult_dsp48e_yy_5/1(c_re) -> y5y5*/1
  cmult_dsp48e_xx_5/1(c_re) -> x5x5*/1
  y5/1 -> c_to_ri_y_5/1
  x5/1 -> c_to_ri_x_5/1
  cmult_dsp48e_xy_4/2(c_im) -> x4y4*_im/1
  cmult_dsp48e_xy_4/1(c_re) -> x4y4*_re/1
  cmult_dsp48e_yy_4/1(c_re) -> y4y4*/1
  cmult_dsp48e_xx_4/1(c_re) -> x4x4*/1
  y4/1 -> c_to_ri_y_4/1
  x4/1 -> c_to_ri_x_4/1
  cmult_dsp48e_xy_3/2(c_im) -> x3y3*_im/1
  cmult_dsp48e_xy_3/1(c_re) -> x3y3*_re/1
  cmult_dsp48e_yy_3/1(c_re) -> y3y3*/1
  cmult_dsp48e_xx_3/1(c_re) -> x3x3*/1
  y3/1 -> c_to_ri_y_3/1
  x3/1 -> c_to_ri_x_3/1
  cmult_dsp48e_xy_2/2(c_im) -> x2y2*_im/1
  cmult_dsp48e_xy_2/1(c_re) -> x2y2*_re/1
  cmult_dsp48e_yy_2/1(c_re) -> y2y2*/1
  cmult_dsp48e_xx_2/1(c_re) -> x2x2*/1
  y2/1 -> c_to_ri_y_2/1
  x2/1 -> c_to_ri_x_2/1
  cmult_dsp48e_xy_1/2(c_im) -> x1y1*_im/1
  cmult_dsp48e_xy_1/1(c_re) -> x1y1*_re/1
  cmult_dsp48e_yy_1/1(c_re) -> y1y1*/1
  cmult_dsp48e_xx_1/1(c_re) -> x1x1*/1
  y1/1 -> c_to_ri_y_1/1
  x1/1 -> c_to_ri_x_1/1
  cmult_dsp48e_xy_0/2(c_im) -> x0y0*_im/1
  cmult_dsp48e_xy_0/1(c_re) -> x0y0*_re/1
  cmult_dsp48e_yy_0/1(c_re) -> y0y0*/1
  cmult_dsp48e_xx_0/1(c_re) -> x0x0*/1
  y0/1 -> c_to_ri_y_0/1
  x0/1 -> c_to_ri_x_0/1

== system h16k_ver112c_1500/Subsystem ==
  In2 : Inport
  Register{3..8,14..15,17,21,23..24,26..37} (24 alike) : xbsIndex_r4/Register  init=0  rst=off  en=off  dbl_ovrd=off  block_type=register
      settings: block_version=11.4
  Out1 : Outport
  Out2 : Outport  Port=2
  Out3 : Outport  Port=3
  Out4 : Outport  Port=4
  wires:
  Register7/1 -> Register6/1
  Register6/1 -> Register3/1
  Register8/1 -> Register5/1
  Register5/1 -> Register4/1
  Register3/1 -> Register8/1
  Register23/1 -> Register21/1
  Register21/1 -> Register14/1
  Register24/1 -> Register17/1
  Register17/1 -> Register15/1
  Register14/1 -> Register24/1
  Register30/1 -> Register29/1
  Register29/1 -> Register26/1
  Register31/1 -> Register28/1
  Register28/1 -> Register27/1
  Register26/1 -> Register31/1
  Register36/1 -> Register35/1
  Register35/1 -> Register32/1
  Register37/1 -> Register34/1
  Register34/1 -> Register33/1
  Register32/1 -> Register37/1
  In2/1 -> Register36/1, Register30/1, Register23/1, Register7/1
  Register4/1 -> Out1/1
  Register15/1 -> Out2/1
  Register27/1 -> Out3/1
  Register33/1 -> Out4/1
